simulink library "aeroblk_lib_HL20"  (R2023a)
settings: Solver=ode45  StartTime=0.0  StopTime=10.0  RelTol=1e-3
values from neighbouring files (symbols this model uses):
  alpha_vec_Cn0 = [-10 -5 0 5 10 15 20 25 30]    [aeroblk_init_HL20.m]
  b_ref = 13.89/m2ft    (= 4.23367186452)    [aeroblk_init_HL20.m]
  beta_vec_Cn0 = [0 2 5 10]    [aeroblk_init_HL20.m]
  Clbeta = -0.00787    [aeroblk_init_HL20.m]
  Clda = temp(:,6)    [aeroblk_init_HL20.m]
  Clddf = temp(:,4)    [aeroblk_init_HL20.m]
  Cldr = temp(:,6)    [aeroblk_init_HL20.m]
  Clp = [-4.98 -6.0 -3.98 -5.79 -4.25 -4.99 -6.49 -6.19 -8.10 -8.72 -24.10]*1e-1    [aeroblk_init_HL20.m]
  Clr = [4.96 5.98 8.40 8.06 6.86 5.72 6.03 8.99 9.57 13.57 44.90]*1e-1    [aeroblk_init_HL20.m]
  Cm0 = reshape(temp(:,2),length(beta_vec_0),length(alpha_vec_0))    [aeroblk_init_HL20.m]
  Cmda = temp(:,2)    [aeroblk_init_HL20.m]
  Cmde = temp(:,2)    [aeroblk_init_HL20.m]
  Cmdfn = temp(:,2)    [aeroblk_init_HL20.m]
  Cmdfp = temp(:,2)    [aeroblk_init_HL20.m]
  Cmdr = temp(:,2)    [aeroblk_init_HL20.m]
  Cmq = [-2.03 -1.58 -1.16 -1.76 -1.76 -1.75 -1.74 -2.52 -2.99 -5.71 -8]*1e-1    [aeroblk_init_HL20.m]
  Cn0 = [0 0.46 1.15 2.30 ... (first row only)    [aeroblk_init_HL20.m]
  Cnda = temp(:,5)    [aeroblk_init_HL20.m]
  Cnddf = temp(:,3)    [aeroblk_init_HL20.m]
  Cndr = temp(:,5)    [aeroblk_init_HL20.m]
  Cnp = [3.81 3.53 2.19 2.44 1.79 1.67 2.01 2.22 3.07 3.79 8.50]*1e-1    [aeroblk_init_HL20.m]
  Cnr = [-7.94 -8.37 -9.21 -9.22 -8.67 -9.22 -9.46 -10.07 -10.90 -12.86 -20.41]*1e-1    [aeroblk_init_HL20.m]
  CX0 = -reshape(temp(:,3),length(beta_vec_0),length(alpha_vec_0))    [aeroblk_init_HL20.m]
  CXda = -temp(:,3)    [aeroblk_init_HL20.m]
  CXddf = temp(:,1)    [aeroblk_init_HL20.m]
  CXde = -temp(:,3)    [aeroblk_init_HL20.m]
  CXdfn = -temp(:,3)    [aeroblk_init_HL20.m]
  CXdfp = -temp(:,3)    [aeroblk_init_HL20.m]
  CXdr = -temp(:,3)    [aeroblk_init_HL20.m]
  CYbeta = -0.01242    [aeroblk_init_HL20.m]
  CYda = temp(:,4)    [aeroblk_init_HL20.m]
  CYddf = temp(:,2)    [aeroblk_init_HL20.m]
  CYdr = temp(:,4)    [aeroblk_init_HL20.m]
  CZ0 = -reshape(temp(:,1),length(beta_vec_0),length(alpha_vec_0))    [aeroblk_init_HL20.m]
  CZda = -temp(:,1)    [aeroblk_init_HL20.m]
  CZde = -temp(:,1)    [aeroblk_init_HL20.m]
  CZdfn = -temp(:,1)    [aeroblk_init_HL20.m]
  CZdfp = -temp(:,1)    [aeroblk_init_HL20.m]
  CZdr = -temp(:,1)    [aeroblk_init_HL20.m]
  d_ref = 28.24/m2ft    (= 8.60755172456)    [aeroblk_init_HL20.m]
  mass = massBody+massFuel    (= 11738.9844962)    [aeroblk_init_HL20.m]
  x_cg = 0.575*len_veh    (= 4.78635044684)    [aeroblk_init_HL20.m]
  x_ref = 0.54*len_veh    (= 4.49500737616)    [aeroblk_init_HL20.m]
undefined symbols (not defined in the file or in its folder): a_matrix, A_matrix, b_matrix, B_matrix, c_matrix, C_matrix, d_matrix, F, F_matrix, H_matrix, Kalpha, Kalpha_1, Kbeta, Kbeta_1, Kp, Kp_1, Kphi, Kphi_1, Kq, Kq_1, Kr, Kr_1, Light, MIL
libraries: aerolibschedule x4, aerolibconvert2 x3, aerolibasang x3, aerolibwind2 x3, shared6dof x1, aerolibatmos2 x1, aerolibadyn x1
(part 2 of 2)

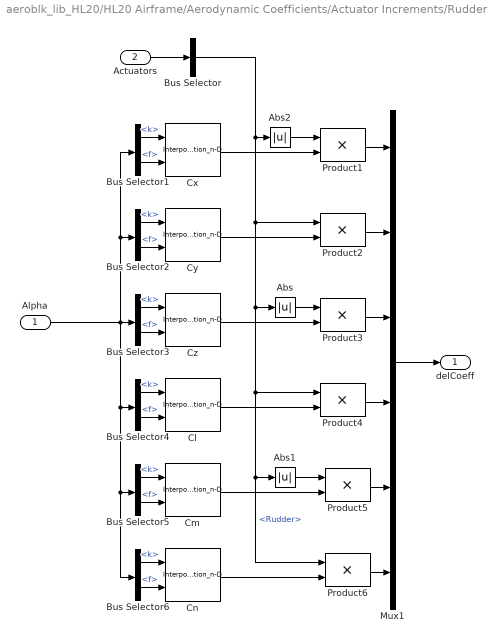
== system aeroblk_lib_HL20/HL20 Airframe/Aerodynamic Coefficients/Actuator Increments/Rudder ==
  Alpha : Inport
  Actuators : Inport  Port=2
  Abs : Abs
  Abs1 : Abs
  Abs2 : Abs
  Bus Selector : BusSelector  OutputSignals=Rudder
  Bus Selector{1..6} (6 alike) : BusSelector  OutputSignals=k,f
  Cl : Interpolation_n-D  NumberOfTableDimensions=1  Table=Cldr  RemoveProtectionIndex=on
      settings: InputPortMap=u0,u1
  Cm : Interpolation_n-D  NumberOfTableDimensions=1  Table=Cmdr  RemoveProtectionIndex=on
      settings: InputPortMap=u0,u1
  Cn : Interpolation_n-D  NumberOfTableDimensions=1  Table=Cndr  RemoveProtectionIndex=on
      settings: InputPortMap=u0,u1
  Cx : Interpolation_n-D  NumberOfTableDimensions=1  Table=CXdr  RemoveProtectionIndex=on
      settings: InputPortMap=u0,u1
  Cy : Interpolation_n-D  NumberOfTableDimensions=1  Table=CYdr  RemoveProtectionIndex=on
      settings: InputPortMap=u0,u1
  Cz : Interpolation_n-D  NumberOfTableDimensions=1  Table=CZdr  RemoveProtectionIndex=on
      settings: InputPortMap=u0,u1
  Mux1 : Mux  Inputs=6
  Product{1..6} (6 alike) : Product  InputSameDT=on  SaturateOnIntegerOverflow=on  OutDataTypeStr=Inherit: Same as first input
  delCoeff : Outport  VectorParamsAs1DForOutWhenUnconnected=off
  wires:
  Actuators/1 -> Bus Selector/1
  Mux1/1 -> delCoeff/1
  Product1/1 -> Mux1/1
  Cx/1 -> Product1/2
  Product2/1 -> Mux1/2
  Cy/1 -> Product2/2
  Product3/1 -> Mux1/3
  Cz/1 -> Product3/2
  Cl/1 -> Product4/2
  Product4/1 -> Mux1/4
  Cm/1 -> Product5/2
  Product5/1 -> Mux1/5
  Cn/1 -> Product6/2
  Product6/1 -> Mux1/6
  Bus Selector/1 -> Abs2/1, Product2/1, Abs/1, Product4/1, Abs1/1, Product6/1  "<Rudder>"
  Abs/1 -> Product3/1
  Abs1/1 -> Product5/1
  Abs2/1 -> Product1/1
  Alpha/1 -> Bus Selector3/1, Bus Selector4/1, Bus Selector6/1, Bus Selector5/1, Bus Selector2/1, Bus Selector1/1
  Bus Selector1/1 -> Cx/1  "<k>"
  Bus Selector1/2 -> Cx/2  "<f>"
  Bus Selector2/1 -> Cy/1  "<k>"
  Bus Selector2/2 -> Cy/2  "<f>"
  Bus Selector3/1 -> Cz/1  "<k>"
  Bus Selector3/2 -> Cz/2  "<f>"
  Bus Selector4/1 -> Cl/1  "<k>"
  Bus Selector4/2 -> Cl/2  "<f>"
  Bus Selector5/1 -> Cm/1  "<k>"
  Bus Selector5/2 -> Cm/2  "<f>"
  Bus Selector6/1 -> Cn/1  "<k>"
  Bus Selector6/2 -> Cn/2  "<f>"

== system aeroblk_lib_HL20/HL20 Airframe/Aerodynamic Coefficients/Body Rate Damping/p ==
  Alpha : Inport
  Bus Selector : BusSelector  OutputSignals=k,f
  Bus Selector1 : BusSelector  OutputSignals=k,f
  Cl : Interpolation_n-D  NumberOfTableDimensions=1  Table=Clp  RemoveProtectionIndex=on
      settings: InputPortMap=u0,u1
  Cn : Interpolation_n-D  NumberOfTableDimensions=1  Table=Cnp  RemoveProtectionIndex=on
      settings: InputPortMap=u0,u1
  Constant1 : Constant  Value=0
  Mux1 : Mux  Inputs=6
  delCoeff : Outport  VectorParamsAs1DForOutWhenUnconnected=off
  wires:
  Mux1/1 -> delCoeff/1
  Constant1/1 -> Mux1/1, Mux1/5, Mux1/3, Mux1/2  "Cxp"
  Cn/1 -> Mux1/6
  Cl/1 -> Mux1/4  "Cl"
  Alpha/1 -> Bus Selector/1, Bus Selector1/1
  Bus Selector/1 -> Cl/1  "<k>"
  Bus Selector/2 -> Cl/2  "<f>"
  Bus Selector1/1 -> Cn/1  "<k>"
  Bus Selector1/2 -> Cn/2  "<f>"

== system aeroblk_lib_HL20/HL20 Airframe/Aerodynamic Coefficients/Body Rate Damping/q ==
  Alpha : Inport
  Bus Selector1 : BusSelector  OutputSignals=k,f
  Cmq : Interpolation_n-D  NumberOfTableDimensions=1  Table=Cmq  RemoveProtectionIndex=on
      settings: InputPortMap=u0,u1
  Constant3 : Constant  Value=0
  Mux1 : Mux  Inputs=6
  delCoeff : Outport  VectorParamsAs1DForOutWhenUnconnected=off
  wires:
  Cmq/1 -> Mux1/5
  Constant3/1 -> Mux1/1, Mux1/2, Mux1/3, Mux1/6, Mux1/4
  Mux1/1 -> delCoeff/1
  Alpha/1 -> Bus Selector1/1
  Bus Selector1/1 -> Cmq/1  "<k>"
  Bus Selector1/2 -> Cmq/2  "<f>"

== system aeroblk_lib_HL20/HL20 Airframe/Aerodynamic Coefficients/Body Rate Damping/r ==
  Alpha : Inport
  Bus Selector : BusSelector  OutputSignals=k,f
  Bus Selector1 : BusSelector  OutputSignals=k,f
  Cl : Interpolation_n-D  NumberOfTableDimensions=1  Table=Clr  RemoveProtectionIndex=on
      settings: InputPortMap=u0,u1
  Cn : Interpolation_n-D  NumberOfTableDimensions=1  Table=Cnr  RemoveProtectionIndex=on
      settings: InputPortMap=u0,u1
  Constant : Constant  Value=0
  Mux1 : Mux  Inputs=6
  delCoeff : Outport  VectorParamsAs1DForOutWhenUnconnected=off
  wires:
  Cn/1 -> Mux1/6
  Cl/1 -> Mux1/4  "Cl"
  Constant/1 -> Mux1/1, Mux1/2, Mux1/5, Mux1/3  "Cxr"
  Mux1/1 -> delCoeff/1
  Alpha/1 -> Bus Selector1/1, Bus Selector/1
  Bus Selector/1 -> Cl/1  "<k>"
  Bus Selector/2 -> Cl/2  "<f>"
  Bus Selector1/1 -> Cn/1  "<k>"
  Bus Selector1/2 -> Cn/2  "<f>"
